simulink model "AAA"  (Simulink 6.6)
settings: Solver=FixedStepDiscrete  StartTime=0.0  StopTime=40  RelTol=1e-3
values from neighbouring files (symbols this model uses):
  Kp = 50*eye(3)    [ex_robot.m]
  manip3 = manipulator(DHantrosph,'manip3',Tb0,Tne)    [ex_num_anthrop_sph_wrist.m]
  Ts_mdl = 0.01    [ex_robot.m]
libraries: DAMA_lib x8, vrlib x1
settings Model: Creator=dario  LastModifiedBy=mofo  ExtModeAutoUpdateStatusClock=off

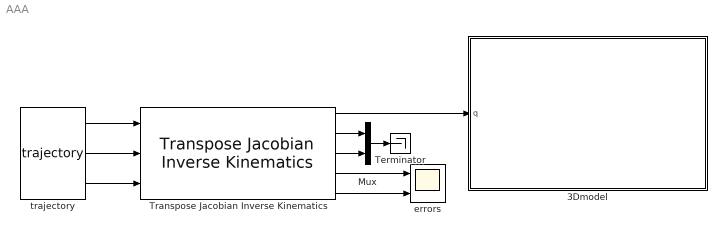
== system AAA ==
  3Dmodel : Subsystem  AncestorBlock=DAMA_lib/3D/3Dmodel  mask(3D model){sel_obj_nam=Manipulator Name, robot=manip3, wrlfile=manipVR_base.wrl, SampleTime=Ts_mdl, show_ax=off, show_3D_param=off, CaptureFileFormat=png, CaptureFileName='%f_shot_%n.png', Record3D=off, Record3DFileName='%f_anim_%n.wrl', Record2D=off, Record2DCompressMethod=none, Record2DFPS=15, Record2DFileName='%f_anim_%n.avi', Wireframe=off, Viewpoint=STD, RecordMode=scheduled, RecordInterval=[0 10]}
      mask prompts: sel_obj_nam "Input Method"; robot "Manipulator Name"; wrlfile "WRL file name"; SampleTime "3D Sample Time"; show_ax "enable "show axes" input"; show_3D_param "show VRML parameters"; CaptureFileFormat "screenshot file format"; CaptureFileName "screenshot file name (string)"; Record3D "RecordWRL"; Record3DFileName "WRL file name (string)"; Record2D "Record AVI"; Record2DCompressMethod "AVI Compression"; Record2DFPS "AVI FPS"; Record2DFileName "AVI file name (string)"; RecordInterval "Record Interval"
      mask help:
      | Display the 3D model associated with a manipulator.
      |
      | Block Inputs:
      | 1st: signal with joint positions
      | 2nd (if enabled): logical input, if true show frame-axes in 3D animation.
      |
      | Copyright (C) 2009, by Carmine Dario Bellicoso and Marco Caputano.
      | This file is part of DAMA^{ROB} v.???
      | relased under GNU license LGPLv2.1
      mask init:
      | %% SOME INIT
      | mainblock = gcb;
      | blocks = get(gcbh,'Blocks');
      | load_system('DAMA_lib');
      | VR_handle = get_param([gcb,'/VR'],'Handle');
      | % StartTime = str2num(get_param(gcs,'StartTime'));
      | 
      | if strcmp(get_param(gcs,'SimulationStatus'),'stopped')  % operate inside the block only simulation is not running
      |     %% there's something inside the block, delete everything but the inport and VR!
      |     if length(blocks) >= 2
      |         lin = get_param(mainblock,'lines');     % delete lines
      |         if ~isempty(lin)
      |             delete(lin.Handle);
      |         end
      |         for i = 2:1:length(blocks)              % delete blocks
      |             if strcmp(blocks{i},'VR') ~= 1
      |                 delete_block([mainblock,'/',blocks{i}])
      |             end
      |         end
      |         set_param(mainblock,'MaskDisplay', 'disp(''select manipulator'')' );    % change mask aspect
      |         orig_pos = get_param(mainblock,'Position');
      |         new_pos = orig_pos([1,2,1,2]) + [ 0 0 170 65];
      |         set_param(mainblock,'Position', new_pos);
      |     end
      | 
      | 
      |     %% extract information from input data (oject name / WRL file)
      |     if strcmp(sel_obj_nam,'Manipulator Name')
      |         if isa( robot, 'manipulator') && (robot.DH.r ~= 0)
      |             robot_name = robot.name;
      |             DH = robot.DH.table;
      |             r = size(DH)*[1;0];
      |             wrlfile = [robot_name,'VR_base.wrl'];
      |             imagefile = [robot_name,'_3D.png'];
      |         else
      |             return
      |         end
      |     else
      |         if strcmp(sel_obj_nam,'WRL file name')           % WRL file
      |             if exist(wrlfile,'file')
      |                 robot_name = wrlfile(1:end-11);
      |                 imagefile = [robot_name,'_3D.png'];
      |                 f = fopen(wrlfile,'r');
      |                 DH5 = fgetl(f);  %#ok<NASGU>
      |                 DH5 = fgetl(f);
      |                 DH5 = DH5(11:end);
      |                 fclose(f);
      |                 DH5n = eval(DH5);
      |                 r = length(DH5n);
      |                 DH(:,5) = DH5n;
      |             else
      |                 return
      |             end
      |         end
      |     end
      | 
      |     %% specified manipulator or WRL file exists, let's create the subsystem!
      |     if ~exist(imagefile,'file')
      |         imagefile = 'dama_150.png';
      |     end
      |     png = imread(imagefile);
      |     dimY_png = size(png)*[1; 0; 0];
      |     dimX_png = size(png)*[0; 1; 0];
      |     if dimY_png >= 150
      |         dimY = 150;
      |         dimX = round(dimY * dimX_png/dimY_png);
      |     else
      |         dimY = dimY_png;
      |         dimX = dimX_png;
      |     end
      |     Mask_Disp_string = ['image(imread(''',imagefile,'''))',';port_label(''input'',1,''q'');'];
      |     nodes = '';         % VRML nodes to modify
      |     for i = 1:1:r
      |         if DH(i,5) == 0
      |             nodes = [nodes, 'Z', num2str(i-1) ,'.rotation.4.1.double#' ];  %#ok<AGROW>
      |         else
      |             nodes = [nodes, 'Link',num2str(i),'.translation.3#' ];  %#ok<AGROW>
      |         end
      |     end
      | 
      |     for i = 1:1:r
      |         nodes = [nodes,'Xaxis',num2str(i-1),'.scale#']; %#ok<AGROW>
      |         nodes = [nodes,'Yaxis',num2str(i-1),'.scale#']; %#ok<AGROW>
      |         nodes = [nodes,'Zaxis',num2str(i-1),'.scale#']; %#ok<AGROW>
      |     end
      |     nodes = nodes(1:end-1);
      | 
      |     % add demux and connect input 'q' to it
      |     add_block('built-in/demux', [mainblock,'/demux'],...
      |         'DisplayOption','bar',...
      |         'Position','[90,29,95,211]',...
      |         'ShowName','off',...
      |         'Outputs',num2str(r));
      |     add_line(mainblock,'q/1','demux/1');
      | 
      |     % modify VR sink
      |     set_param([mainblock,'/VR'],...
      |         'Position','[360,69,455,141]',...
      |         'WorldFileName',wrlfile,...
      |         'WorldDescription',['3DAMA manipulator: ',robot_name],...
      |         'AutoView','off',...
      |         'SampleTime',num2str(SampleTime),...
      |         'FieldsWritten',nodes, ...
      |         'FigureProperties', '{''Position'', ''Name'', ''Viewpoint'', ''CameraBound'', ''CameraDirection'', ''CameraPosition'', ''CameraUpVector'', ''ZoomFactor'', ''Antialiasing'', ''Headlight'', ''Lighting'', ''NavPanel'', ''StatusBar'', ''ToolBar'', ''Textures'', ''Transparency'', ''Wireframe'', ''NavZones'', ''NavMode'', ''NavSpeed'', ''Record2DCompressMethod'', ''Record2DCompressQuality'', ''Record2D'', ''Record2DFileName'', ''Record2DFPS'';                [5.0000000000000000e+00   9.7000000000000000e+01   7.8400000000000000e+02   5.3800000000000000e+02], ''scara'', ''_untitled_1'', ''on'', [-1.9898756659875949e-02   1.7901367086524811e-01  -9.8364533503023699e-01], [8.8076866149981403e-01  -7.9236092358681276e+00  -7.2561079645852544e-01], [1.9965352243806467e-03   9.8384528836631602e-01   1.7900967126522893e-01], [1.0000000000000000e+00], ''on'', ''on'', ''on'', ''halfbar'', ''on'', ''on'', ''on'', ''on'', ''off'', ''off'', ''examine'', ''normal'', ''auto'', [7.5000000000000000e+01], ''on'', ''%f_anim2_%n.avi'', [1.0000000000000000e+01]}' );
      | 
      |     % add VR rotation and VR translation blocks, with offset and connections
      |     for i = 1:1:length( DH(:,5) )
      |         position = [200, 50, 270, 80] + [0 50 0 50]*(i-1);
      |         if DH(i,5) == 0
      |             add_block('DAMA_lib/util/rotation', [mainblock,'/rotation',num2str(i)]);
      |             set_param([mainblock,'/rotation',num2str(i)],'Position',position);
      |             add_block('built-in/constant', [mainblock,'/offset',num2str(i)]);
      |             set_param([mainblock,'/offset',num2str(i)],'Value','0');                                         % OFFSET HERE
      |             set_param([mainblock,'/offset',num2str(i)],'Position',position - [65,-18,95,-2]);
      |             add_line(mainblock,['rotation',num2str(i),'/1'], ['VR/',num2str(i)]);
      |             add_line(mainblock,['offset',num2str(i),'/1'],['rotation',num2str(i),'/2']);
      |             add_line(mainblock,['demux/',num2str(i)],['rotation',num2str(i),'/1']);
      |         else
      |             add_block('DAMA_lib/util/translation', [mainblock,'/translation',num2str(i)]);
      |             set_param([mainblock,'/translation',num2str(i)],'Position',position);
      |             add_block('built-in/constant', [mainblock,'/offset',num2str(i)]);
      |             set_param([mainblock,'/offset',num2str(i)],'Value','0.5');                                         % OFFSET HERE
      |             set_param([mainblock,'/offset',num2str(i)],'Position',position - [65,-18,95,-2]);
      |             add_line(mainblock,['translation',num2str(i),'/1'], ['VR/',num2str(i)]);
      |             add_line(mainblock,['offset',num2str(i),'/1'],['translation',num2str(i),'/2']);
      |             add_line(mainblock,['demux/',num2str(i)],['translation',num2str(i),'/1']);
      |         end
      |     end
      | 
      |     % add scale control for axes
      |     add_block('built-in/Product',[mainblock,'/show'],...
      |         'Position',[435,212,475,248]);
      |     add_block('built-in/Constant',[mainblock,'/scale'],...
      |         'Value','[1,1,1]',...
      |         'Position','[370,232,410,248]');
      |     add_line(mainblock,'scale/1','show/2');
      |     for i=r+1:1:r+(3*r)
      |         add_line(mainblock,'show/1',['VR/',num2str(i)]);
      |     end
      | 
      |     % inport 2 or constant '1'
      |     if strcmp(get_param(mainblock,'show_ax'),'on')
      |         add_block('built-in/Inport',[mainblock,'/axes_en'],...
      |             'Position','[375,203,405,217]');
      |         Mask_Disp_string = [Mask_Disp_string ,';port_label(''input'',2,''axes'');'];
      |     else
      |         add_block('built-in/Constant',[mainblock,'/axes_en'],...
      |             'Value','1',...
      |             'Position','[375,203,405,217]');
      |     end
      |     add_line(mainblock,'axes_en/1','show/1');
      | 
      |     % change mask aspect
      |     set_param(mainblock,'MaskDisplay',Mask_Disp_string);
      |     orig_pos = get_param(mainblock,'Position');
      |     new_pos = orig_pos([1,2,1,2]) + [ 0 0 dimX dimY];
      |     set_param(mainblock,'Position', new_pos);
      | 
      |     % add 'show 3D' block
      |     %     add_block('DAMA_lib/util/show_3D', [mainblock,'/Show_3D'], ...
      |     %         'Position','[375,286,448,316]');
      | 
      |     vrmfunc('FnOpen', VR_handle );
      |     try
      |         wrl_file = get(get_param([mainblock,'/VR'],'Handle'),'WorldFileName');
      |         list_world_corresp = strfind(get(vrworld(vrsfunc('VRT3ListScenes')),'FileName'),wrl_file);
      |         if length(list_world_corresp) == 1
      |             num_world_found = 1;
      |         else
      |             for i=1:length(list_world_corresp)
      |                 if ~isempty(list_world_corresp{i})
      |                     num_world_found = i;
      |                     break
      |                 end
      |             end
      |         end
      |         ls_wrworlds = vrwho;
      | 
      |         w = ls_wrworlds(num_world_found);
      |         f = get(w, 'Figures');
      |     catch
      |         w = vrworld;
      |         f = vrfigure;
      |     end
      | 
      |     if isvalid(w)
      |         if RecordMode == 1
      |             set(w,'RecordMode','manual');
      |         else
      |             set(w,'RecordMode','scheduled');
      |         end
      |         set(w,'RecordInterval', RecordInterval);
      | 
      |         if Record3D == 0
      |             set(w,'Record3D','off');
      |         else
      |             set(w,'Record3D','on');
      |         end
      |         set(w,'Record3DFileName',Record3DFileName);
      |     end
      | 
      |     if isvalid(f)
      |         if CaptureFileFormat == 1
      |             set(f,'CaptureFileFormat','png');
      |         else
      |             set(f,'CaptureFileFormat','tif');
      |         end
      | 
      |         if Record2D == 0
      |             set(f,'Record2D','off');
      |         else
      |             set(f,'Record2D','on');
      |         end
      | 
      |         if Record2DCompressMethod == 1
      |             set(f,'Record2DCompressMethod','none');
      |         else
      |             set(f,'Record2DCompressMethod','auto');
      |         end
      | 
      |         if Wireframe == 0
      |             set(f,'Wireframe','off');
      |         else
      |             set(f,'Wireframe','on');
      |         end
      | 
      |         if Viewpoint == 1
      |             set(f,'Viewpoint','STD');
      |         elseif Viewpoint == 2
      |             set(f,'Viewpoint','XY_plane');
      |         elseif Viewpoint == 3
      |             set(f,'Viewpoint','XY_perspective');
      |         elseif Viewpoint == 4
      |             set(f,'Viewpoint','left view (XZ)');
      |         elseif Viewpoint == 5
      |             set(f,'Viewpoint','right view (-XZ)');
      |         elseif Viewpoint == 6
      |             set(f,'Viewpoint','rear view (-YZ)');
      |         elseif Viewpoint == 7
      |             set(f,'Viewpoint','front view (-YZ)');
      |         end
      | 
      |         set(f,'Record2DFPS',Record2DFPS);
      |         set(f,'CaptureFileName',CaptureFileName);
      |         set(f,'Record2DFileName',Record2DFileName);
      |     end
      | 
      | else
      | 
      |     try
      |         wrl_file = get(get_param([mainblock,'/VR'],'Handle'),'WorldFileName');
      |         list_world_corresp = strfind(get(vrworld(vrsfunc('VRT3ListScenes')),'FileName'),wrl_file);
      |         if length(list_world_corresp) == 1
      |             num_world_found = 1;
      |         else
      |             for i=1:length(list_world_corresp)
      |                 if ~isempty(list_world_corresp{i})
      |                     num_world_found = i;
      |                     break
      |                 end
      |             end
      |         end
      |         ls_wrworlds = vrwho;
      | 
      |         w = ls_wrworlds(num_world_found);
      |         f = get(w, 'Figures');
      |         if isempty(f)
      |             vrmfunc('FnOpen', VR_handle );
      |         end
      |     catch
      |         w = vrworld;
      |         f = vrfigure;
      |     end
      | 
      |     if isvalid(w)
      |         if RecordMode == 1
      |             set(w,'RecordMode','manual');
      |         else
      |             set(w,'RecordMode','scheduled');
      |         end
      |         set(w,'RecordInterval', RecordInterval);
      | 
      |         if Record3D == 0
      |             set(w,'Record3D','off');
      |         else
      |             set(w,'Record3D','on');
      |         end
      |         set(w,'Record3DFileName',Record3DFileName);
      |     end
      | 
      |     if isvalid(f)
      |         if CaptureFileFormat == 1
      |             set(f,'CaptureFileFormat','png');
      |         else
      |             set(f,'CaptureFileFormat','tif');
      |         end
      | 
      |         if Record2D == 0
      |             set(f,'Record2D','off');
      |         else
      |             set(f,'Record2D','on');
      |         end
      | 
      |         if Record2DCompressMethod == 1
      |             set(f,'Record2DCompressMethod','none');
      |         else
      |             set(f,'Record2DCompressMethod','auto');
      |         end
      | 
      |         if Wireframe == 0
      |             set(f,'Wireframe','off');
      |         else
      |             set(f,'Wireframe','on');
      |         end
      | 
      |         if Viewpoint == 1
      |             set(f,'Viewpoint','STD');
      |         elseif Viewpoint == 2
      |             set(f,'Viewpoint','XY_plane');
      |         elseif Viewpoint == 3
      |             set(f,'Viewpoint','XY_perspective');
      |         elseif Viewpoint == 4
      |             set(f,'Viewpoint','left view (XZ)');
      |         elseif Viewpoint == 5
      |             set(f,'Viewpoint','right view (-XZ)');
      |         elseif Viewpoint == 6
      |             set(f,'Viewpoint','rear view (-YZ)');
      |         elseif Viewpoint == 7
      |             set(f,'Viewpoint','front view (-YZ)');
      |         end
      | 
      |         set(f,'Record2DFPS',Record2DFPS);
      |         set(f,'CaptureFileName',CaptureFileName);
      |         set(f,'Record2DFileName',Record2DFileName);
      |     end
      | end
      mask StyleString: popup(Manipulator Name|WRL file name),edit,edit,edit,checkbox,checkbox,popup(png|tif),edit,checkbox,edit,checkbox,popup(none|auto),edit,edit,checkbox,popup(STD|XY_plane|XY_perspective|left view (XZ)|right view (-XZ)|rear view (-YZ)|front view (-YZ)),popup(manual|scheduled),edit
      mask CallbackString:
      | maskStr = get_param(gcb,'MaskValues');
      | Mask_Vis_Cell_Param = get_param(gcb,'MaskVisibilities');
      | 
      | if strcmp(maskStr{1},'Manipulator Name')
      |     Mask_Vis_Cell_Param{2} = 'on';
      |     Mask_Vis_Cell_Param{3} = 'off';
      | else
      |     Mask_Vis_Cell_Param{2} = 'off';
      |     Mask_Vis_Cell_Param{3} = 'on';
      | end
      | 
      | set_param(gcb,'MaskVisibilities', Mask_Vis_Cell_Param);
      | clear maskStr Mask_Vis_Cell_Param|if strcmp(get_param(gcb,'sel_obj_nam'),'Manipulator Name')
      |     manip_name_param = get_param(gcb,'robot');
      |     if exist(manip_name_param,'var') && isa( eval(manip_name_param), 'manipulator')
      |         % do nothing
      |     else
      |         warndlg([manip_name_param,' is not a valid manipulator name.'])
      |     end
      | end
      | clear manip_name_param|if strcmp(get_param(gcb,'sel_obj_nam'),'WRL file name')
      |     wrl_file_name_param = get_param(gcb,'wrlfile');
      |     if exist(wrl_file_name_param,'file')
      |         % do nothing
      |     else
      |         warndlg([wrl_file_name_param,' does''nt exist.'])
      |     end
      | end
      | clear wrl_file_name_param|||maskStr = get_param(gcb,'MaskValues');
      | Mask_Vis_Cell_Param = get_param(gcb,'MaskVisibilities');
      | 
      | if strcmp(maskStr{6},'on')
      |     for i_mask_par=7:18
      |         Mask_Vis_Cell_Param{i_mask_par} = 'on';
      |     end
      | else
      |     for i_mask_par=7:18
      |         Mask_Vis_Cell_Param{i_mask_par} = 'off';
      |     end
      | end
      | 
      | set_param(gcb,'MaskVisibilities', Mask_Vis_Cell_Param);
      | clear maskStr Mask_Vis_Cell_Param i_mask_par
      | ||||||||||||
      mask Display: image(imread('manip3_3D.png'));port_label('input',1,'q');
  Mux : Mux  Inputs=2
  Terminator : Terminator
  Transpose Jacobian Inverse Kinematics : DAMA_lib/Kinematics/Transpose Jacobian Inverse Kinematics  SystemSampleTime=-1  manip=manip3  Kp=Kp  Ko=Ko  q0=zeros(1,6)  Ts=Ts_mdl
  errors : Scope  NumInputPorts=2
      settings: YMin=-1.38778e-17~0  YMax=0.2~0.05
  trajectory : DAMA_lib/Kinematics/trajectory  SystemSampleTime=-1  path_des=path_des
  wires:
  Transpose Jacobian Inverse Kinematics/1 -> 3Dmodel/1(q)
  Mux/1 -> Terminator/1
  Transpose Jacobian Inverse Kinematics/2 -> Mux/1
  Transpose Jacobian Inverse Kinematics/3 -> Mux/2
  trajectory/1 -> Transpose Jacobian Inverse Kinematics/1
  trajectory/2 -> Transpose Jacobian Inverse Kinematics/2
  trajectory/3 -> Transpose Jacobian Inverse Kinematics/3
  Transpose Jacobian Inverse Kinematics/4 -> errors/1
  Transpose Jacobian Inverse Kinematics/5 -> errors/2

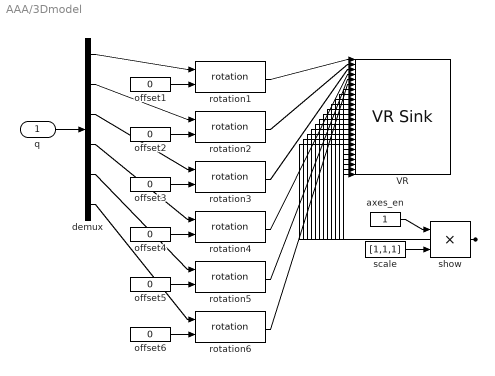
== system AAA/3Dmodel ==
  q : Inport
  VR : vrlib/VR Sink  SampleTime=0.01  ViewEnable=on  RemoteChange=off  RemoteView=on  FieldsWritten=Z0.rotation.4.1.double#Z1.rotation.4.1.double#Z2.rotation.4.1.double#Z3.rotation.4.1.double#Z4.rotation.4.1.double#Z5.rotation.4.1.double#Xaxis0.scale#Yaxis0.scale#Zaxis0.scale#Xaxis1.scale#Yaxis1.scale#Zaxis1.scale#Xaxis2.scale#Yaxis2.scale#Zaxis2.scale#Xaxis3.scale#Yaxis3.scale#Zaxis3.scale#Xaxis4.scale#Yaxis4.scale#Zaxis4.scale#Xaxis5.scale#Yaxis5.scale#Zaxis5.scale  WorldFileName=manip3VR_base.wrl  WorldDescription=3DAMA manipulator: manip3  AutoView=off  FigureProperties="{'Position', 'Name', 'Viewpoint', 'CameraBound', 'CameraDirection', 'CameraPosition', 'CameraUpVector', 'ZoomFactor', 'Antialiasing', 'Headlight', 'Lighting', 'NavPanel', 'StatusBar', 'ToolBar', 'Textures', 'Transparency', 'Wireframe', 'NavZones', 'NavMode', 'NavSpeed', 'Record2DCompressMethod', 'Record2DCompressQuality', 'Record2D', 'Record2DFileName', 'Record2DFPS';                [5.0000000000000000e+00   9.7000000000000000e+01   7.8400000000000000e+02   5.3800000000000000e+02], 'scara', '_untitled_1', 'on', [-1.9898756659875949e-02   1.7901367086524811e-01  -9.8364533503023699e-01], [8.8076866149981403e-01  -7.9236092358681276e+00  -7.2561079645852544e-01], [1.9965352243806467e-03   9.8384528836631602e-01   1.7900967126522893e-01], [1.0000000000000000e+00], 'on', 'on', 'on', 'halfbar', 'on', 'on', 'on', 'on', 'off', 'off', 'examine', 'normal', 'auto', [7.5000000000000000e+01], 'on', '%f_anim2_%n.avi', [1.0000000000000000e+01]}"
  axes_en : Constant
  demux : Demux  Outputs=6
  offset{1..6} (6 alike) : Constant  Value=0
  rotation{1..6} (6 alike) : DAMA_lib/util/rotation  SystemSampleTime=-1
  scale : Constant  Value=[1,1,1]
  show : Product  SaturateOnIntegerOverflow=on  RndMeth=Zero  InputSameDT=on
  wires:
  q/1 -> demux/1
  rotation1/1 -> VR/1
  offset1/1 -> rotation1/2
  demux/1 -> rotation1/1
  rotation2/1 -> VR/2
  offset2/1 -> rotation2/2
  demux/2 -> rotation2/1
  rotation3/1 -> VR/3
  offset3/1 -> rotation3/2
  demux/3 -> rotation3/1
  rotation4/1 -> VR/4
  offset4/1 -> rotation4/2
  demux/4 -> rotation4/1
  rotation5/1 -> VR/5
  offset5/1 -> rotation5/2
  demux/5 -> rotation5/1
  rotation6/1 -> VR/6
  offset6/1 -> rotation6/2
  demux/6 -> rotation6/1
  scale/1 -> show/2
  show/1 -> VR/7, VR/8, VR/9, VR/10, VR/11, VR/12, VR/13, VR/14, VR/15, VR/16, VR/17, VR/18, VR/19, VR/20, VR/21, VR/22, VR/23, VR/24
  axes_en/1 -> show/1
